simulink model "text000"  (Simulink 8.2)
settings: Solver=ode15s  SolverMode=SingleTasking  StartTime=0.0  StopTime=1.5  RelTol=1e-3
values from neighbouring files (symbols this model uses):
  A = [1  2  3  4; 5  6  7  8; 9  10  11  12]    [mytrix.mat]    (also in pisure.m = A + (-1)^(n)*(1/i))
libraries: powerlib x10, powerlib_extras x1
settings Model: Creator=38061  LastModifiedBy=38061  CovMetricSettings=dwe  CovHtmlReporting=off  covSaveCumulativeToWorkspaceVar=off  CovSaveSingleToWorkspaceVar=off  CovExternalEMLEnable=on
settings DataIOCC: LimitDataPoints=off  SaveFormat=StructureWithTime  SignalLoggingSaveFormat=Dataset  ReturnWorkspaceOutputs=on
settings OptimizationCC: ExpressionDepthLimit=128
settings DebuggingCC: UnderspecifiedInitializationDetection=Simplified  MergeDetectMultiDrivingBlocksExec=error  SolverPrmCheckMsg=none  FcnCallInpInsideContextMsg=EnableAllAsError  FrameProcessingCompatibilityMsg=error  StateNameClashWarn=none  SFUnexpectedBacktrackingDiag=error  SFNoUnconditionalDefaultTransitionDiag=error
settings HardwareCC: ProdBitPerPointer=64  ProdLargestAtomicFloat=Float  ProdIntDivRoundTo=Zero  ProdEndianess=LittleEndian  ProdHWDeviceType=Specified
settings ModelReferenceCC: PropagateSignalLabelsOutOfModel=on
settings SFSimCC: SimUseLocalCustomCode=on
settings RTWCC: RTWUseLocalCustomCode=on
settings GRTTargetCC: CodeReplacementLibrary=C99 (ISO)  CombineOutputUpdateFcns=on  GRTInterface=off

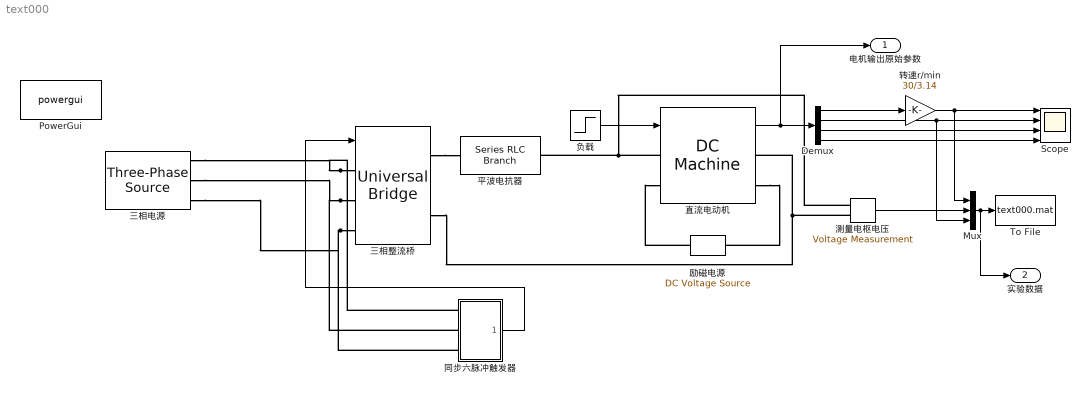
== system text000 ==
  Demux : Demux
  Mux : Mux  Inputs=3
  PowerGui : powerlib/powergui  Priority=1  SimulationMode=Continuous  SampleTime=50e-6  frequency=60  Iterations=50  frequencyindice=50  Pbase=100e6  ErrMax=1e-4  UnitsV=kV  UnitsW=MW  buscounter=0  FunctionMessages=off  echomessages=off  EnableUseOfTLC=off  CurrentSourceSwitches=off  DisableSnubberDevices=off  DisableRonSwitches=off  DisableVfSwitches=off  DisplayEquations=off  AutomaticDiscreteSolvers=off  SolverType=Tustin/Backward Euler (TBE)  Interpol=off  ExternalGateDelay=off  methode=off  Ts=100  x0status=blocks  SPID=on  SwTol=0  HookPort=off  NonlinearTolerance=1e-4  nMaxIteration=100  ContinueOnMaxIteration=off  RestoreLinks=warning  ResistiveCurrentMeasurement=off  Frange=[0:2:500]  Ylog=off  Xlog=on  ShowGrid=off  save=off  variable=ZData  structure=0  ZoomFFT=off  StartTime=0.0  cycles=1  DisplayStyle=1  fundamental=60  FreqAxis=off  MaxFrequency=1000  frequencyindicesteady=1  RmsSteady=1  display=off
  Scope : Scope  NumInputPorts=4
      settings: TimeRange=auto  MaxDataPoints=5000  SaveToWorkspace=off  SaveName=ScopeData  YMin=-35.05567~-5~-5~-5  YMax=330.49762~5~5~5  SampleTime=-1
  To File : ToFile  Filename=text000.mat  SaveFormat=Timeseries
  三相整流桥 : powerlib/Power Electronics/Universal Bridge  Arms=3  SnubberResistance=1e5  SnubberCapacitance=inf  Device=Thyristors  Ron=0.5  Lon=0  ForwardVoltages="[  0  0  ]"  ForwardVoltage=0  GTOparameters=[ 10e-6 , 20e-6 ]  IGBTparameters=[ 1e-6 , 2e-6 ]  Measurements=None  Measurements_2=None  converterType=Rectifier
  三相电源 : powerlib/Electrical Sources/Three-Phase Source  InternalConnection=Yg  VoltagePhases=off  Voltage=142*sqrt(3)  PhaseAngle=0  Voltage_phases=[25e3 25e3 25e3]/sqrt(3)  PhaseAngles_phases=[0 -120 +120]  Frequency=50  NonIdealSource=on  SpecifyImpedance=off  Resistance=0.001  Inductance=0  ShortCircuitLevel=100e6  BaseVoltage=25e3  XRratio=7  BusType=swing  Pref=10e3  Qref=0  Prefabc=[10e3, 10e3, 10e3]  Qrefabc=[0, 0, 0]  Qmin=-inf  Qmax=inf
  励磁电源 : powerlib/Electrical Sources/DC Voltage Source  Amplitude=220  Measurements=None
  同步六脉冲触发器 : Subsystem
  平波电抗器 : powerlib/Elements/Series RLC Branch  LConnTagsString=__new0  RConnTagsString=__new0  BranchType=L  Resistance=0  Inductance=0.02  SetiL0=off  InitialCurrent=0  Capacitance=inf  Setx0=off  InitialVoltage=0  Measurements=None
  测量电枢电压 : powerlib/Measurements/Voltage Measurement  PhasorSimulation=off  OutputType=Complex  PSBequivalent=0
  直流电动机 : powerlib/Machines/DC Machine  PresetModel=No  MechanicalLoad=Torque TL  FieldType=Wound  ShowDetailedParameters=on  MeasurementBus=off  RLa="[ 0.21  0.00021]"  RLf="[ 146.7  0]"  Laf=0.84  MachineConstant=Torque constant (N.m/A)  Ke=1.8  Kt=1.8  J=0.57  Bm=0  Tf=0  w0=1  Ifinit=0.916666666666667  TsPowergui=0  TsBlock=-1
  负载 : Step  Time=0.5  After=171.4  SampleTime=0
  转速r/min : Gain  Gain=30/3.14
  电机输出原始参数 : Outport
  实验数据 : Outport  Port=2
  wires:
  负载/1 -> 直流电动机/1
  直流电动机/1 -> 电机输出原始参数/1, Demux/1
  Demux/3 -> Scope/3
  Demux/4 -> Scope/4
  Demux/2 -> Mux/3, Scope/2
  Demux/1 -> 转速r/min/1
  转速r/min/1 -> Mux/1, Scope/1
  测量电枢电压/1 -> Mux/2
  同步六脉冲触发器/1(pulses) -> 三相整流桥/1
  Mux/1 -> 实验数据/1, To File/1
  connections:
  励磁电源/RConn1 -- 直流电动机/LConn2
  直流电动机/RConn2 -- 励磁电源/LConn1
  三相整流桥/RConn1 -- 平波电抗器/LConn1
  直流电动机/LConn1 -- 测量电枢电压/LConn1 -- 平波电抗器/RConn1
  三相整流桥/RConn2 -- 直流电动机/RConn1 -- 测量电枢电压/LConn2
  三相整流桥/LConn3 -- 同步六脉冲触发器/LConn3 -- 三相电源/RConn3
  三相整流桥/LConn2 -- 同步六脉冲触发器/LConn2 -- 三相电源/RConn2
  三相整流桥/LConn1 -- 同步六脉冲触发器/LConn1 -- 三相电源/RConn1

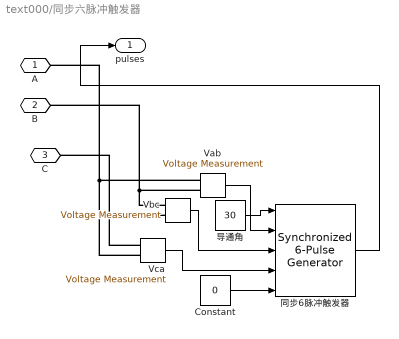
== system text000/同步六脉冲触发器 ==
  Constant : Constant  Value=0
  Vab : powerlib/Measurements/Voltage Measurement  PhasorSimulation=off  OutputType=Complex  PSBequivalent=0
  Vbc : powerlib/Measurements/Voltage Measurement  PhasorSimulation=off  OutputType=Complex  PSBequivalent=0
  Vca : powerlib/Measurements/Voltage Measurement  PhasorSimulation=off  OutputType=Complex  PSBequivalent=0
  同步6脉冲触发器 : powerlib_extras/Control  Blocks/Synchronized 6-Pulse Generator  freq=50  pwidth=10  Double_Pulse=off
  导通角 : Constant  Value=30
  A : PMIOPort  Side=Left
  B : PMIOPort  Port=2  Side=Left
  C : PMIOPort  Port=3  Side=Left
  pulses : Outport
  wires:
  同步6脉冲触发器/1 -> pulses/1
  Vca/1 -> 同步6脉冲触发器/4
  Constant/1 -> 同步6脉冲触发器/5
  导通角/1 -> 同步6脉冲触发器/1
  Vab/1 -> 同步6脉冲触发器/2
  Vbc/1 -> 同步6脉冲触发器/3
  connections:
  Vbc/LConn1 -- B/RConn1 -- Vab/LConn2
  Vca/LConn1 -- C/RConn1 -- Vbc/LConn2
  Vca/LConn2 -- A/RConn1 -- Vab/LConn1
